simulink library "GenericTarget"  (R2025b)
settings: Solver=VariableStepAuto  StartTime=0.0  StopTime=10.0  RelTol=1e-3
undefined symbols (not defined in the file or in its folder): GT_CheckUniqueParameterValue, strlength
libraries: simulink x4, $bdroot x2, etargetslib x1
(part 2 of 3)

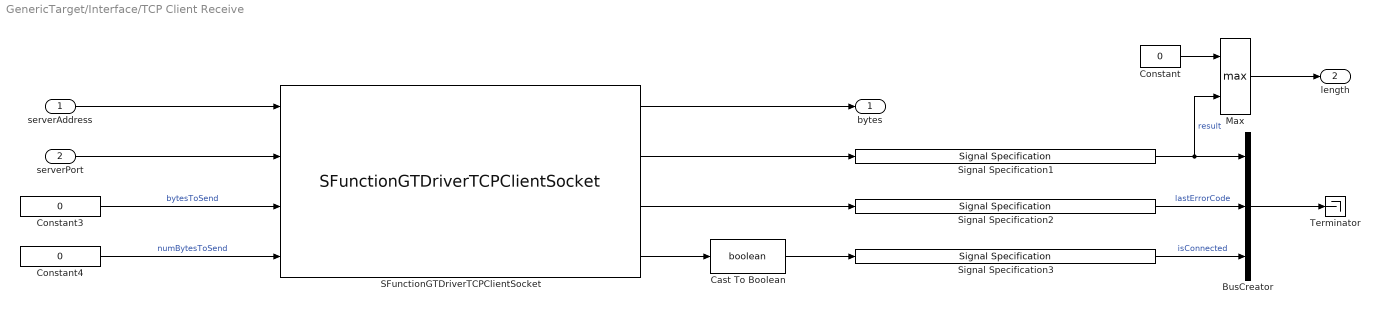
== system GenericTarget/Interface/TCP Client Receive ==
  serverAddress : Inport  OutDataTypeStr=uint8  PortDimensions=4
  serverPort : Inport  Port=2  OutDataTypeStr=uint16  PortDimensions=1
  BusCreator : BusCreator  Inputs=3
  Cast To Boolean : DataTypeConversion  OutDataTypeStr=boolean  SaturateOnIntegerOverflow=off  RndMeth=Floor
  Constant : Constant  Value=0  OutDataTypeStr=int32
  Constant3 : Constant  Value=0  OutDataTypeStr=uint8
  Constant4 : Constant  Value=0  OutDataTypeStr=int32
  Max : MinMax  Function=max  Inputs=2  OutDataTypeStr=int32
  SFunctionGTDriverTCPClientSocket : S-Function  FunctionName=SFunctionGTDriverTCPClientSocket  Parameters=SParameter1, SParameter2, SParameter3, SParameter4, SParameter5, SParameter6, SParameter7, SampleTime  SFunctionDeploymentMode=off  EnableBusSupport=off  mask(Legacy Function){SFunctionSpec=void GT_DriverTCPClientSocketStep(int32 p1, uint8 p5, int32 p6, uint8 y1[p6], int32 y2[1], int32 y3[1], uint8 y4[1], uint8 u1[4], uint16 u2, uint8 p7, uint8 u3[], int32 u4), SParameter1=int32(reshape(localPort, [1 1])), SParameter2=[uint8(deviceName),uint8(0)], SParameter3=uint32(numel(deviceName)), SParameter4=int32(reshape(socketPriority, [1 1])), SParameter5=uint8(0), SParameter6=int32(reshape(rxBufferSize, [1 1])), SParameter7=uint8(reshape(manageConnection, [1 1])), SampleTime=SampleTime, ShowSpec=on}
      mask prompts: SParameter1 "P1:"; SParameter2 "P2:"; SParameter3 "P3:"; SParameter4 "P4:"; SParameter5 "P5:"; SParameter6 "P6:"; SParameter7 "P7:"; SampleTime "Sample time (-1 for inherited):"; ShowSpec "Display function specification"
      mask help:
      | This block allows you to call the legacy functions specified by the following Legacy Code Tool definition:
      | def.SFunctionName = 'SFunctionGTDriverTCPClientSocket';
      | def.OutputFcnSpec = 'void GT_DriverTCPClientSocketStep(int32 p1, uint8 p5, int32 p6, uint8 y1[p6], int32 y2[1], int32 y3[1], uint8 y4[1], uint8 u1[4], uint16 u2, uint8 p7, uint8 u3[], int32 u4)';
      | def.StartFcnSpec = 'void GT_DriverTCPClientSocketInitialize(int32 p1, uint8 p2[], uint32 p3, int32 p4)';
      | def.TerminateFcnSpec = 'void GT_DriverTCPClientSocketTerminate(int32 p1)';
      | def.HeaderFiles = {'GT_DriverTCPClientSocket.hpp'};
      | def.SourceFiles = {'GT_DriverTCPClientSocket.cpp', 'GT_DriverImplementationDetails.cpp'};
      | def.SampleTime = 'parameterized';
      | def.Options.useTlcWithAccel = false;
      | def.Options.language = 'C++';
      mask Help: <p>This block was generated automatically by the Legacy Code Tool. For detailed help on this tool, call<a href="matlab:legacy_code('help')"> legacy_code('help')</a>.</p>
      mask Callback ShowSpec:
      | if strcmp(get_param(gcbh, 'ShowSpec'), 'on')
      |   set_param(gcbh, 'MaskDisplay', sprintf('fprintf(''%s'');', get_param(gcbh, 'SFunctionSpec')));
      | else
      |   set_param(gcbh, 'MaskDisplay', sprintf('fprintf(''%s'');', get_param(gcbh, 'FunctionName')));
      | end
      mask Display: fprintf('void GT_DriverTCPClientSocketStep(int32 p1, uint8 p5, int32 p6, uint8 y1[p6], int32 y2[1], int32 y3[1], uint8 y4[1], uint8 u1[4], uint16 u2, uint8 p7, uint8 u3[], int32 u4)');
  Signal Specification1 : SignalSpecification  OutDataTypeStr=int32  Dimensions=1
  Signal Specification2 : SignalSpecification  OutDataTypeStr=int32  Dimensions=1
  Signal Specification3 : SignalSpecification  OutDataTypeStr=boolean  Dimensions=1
  Terminator : Terminator
  bytes : Outport  OutDataTypeStr=uint8
  length : Outport  Port=2  OutDataTypeStr=int32  PortDimensions=1
  wires:
  Signal Specification2/1 -> BusCreator/2  "lastErrorCode"
  Signal Specification3/1 -> BusCreator/3  "isConnected"
  SFunctionGTDriverTCPClientSocket/1 -> bytes/1
  Constant3/1 -> SFunctionGTDriverTCPClientSocket/3  "bytesToSend"
  Constant4/1 -> SFunctionGTDriverTCPClientSocket/4  "numBytesToSend"
  serverPort/1 -> SFunctionGTDriverTCPClientSocket/2
  serverAddress/1 -> SFunctionGTDriverTCPClientSocket/1
  Cast To Boolean/1 -> Signal Specification3/1
  SFunctionGTDriverTCPClientSocket/2 -> Signal Specification1/1
  SFunctionGTDriverTCPClientSocket/3 -> Signal Specification2/1
  SFunctionGTDriverTCPClientSocket/4 -> Cast To Boolean/1
  Max/1 -> length/1
  Constant/1 -> Max/1
  Signal Specification1/1 -> Max/2, BusCreator/1  "result"
  BusCreator/1 -> Terminator/1

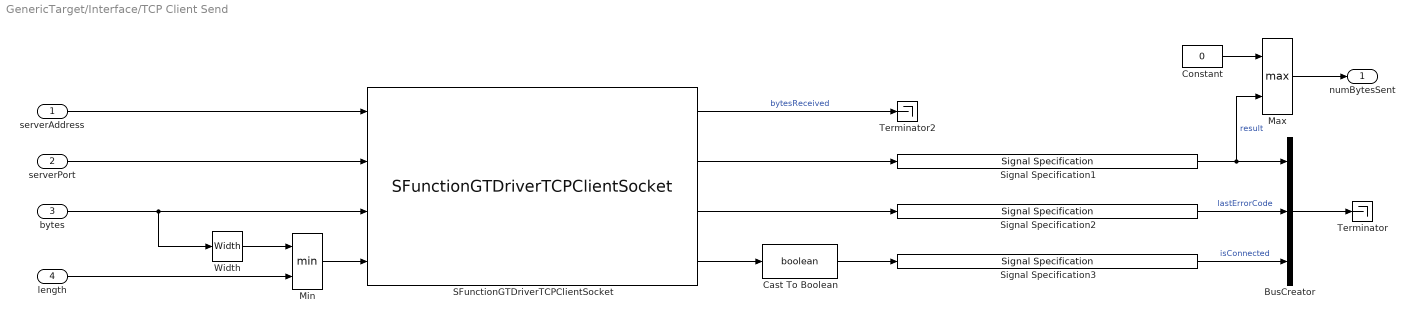
== system GenericTarget/Interface/TCP Client Send ==
  serverAddress : Inport  OutDataTypeStr=uint8  PortDimensions=4
  serverPort : Inport  Port=2  OutDataTypeStr=uint16  PortDimensions=1
  bytes : Inport  Port=3  OutDataTypeStr=uint8
  length : Inport  Port=4  OutDataTypeStr=int32  PortDimensions=1
  BusCreator : BusCreator  Inputs=3
  Cast To Boolean : DataTypeConversion  OutDataTypeStr=boolean  SaturateOnIntegerOverflow=off  RndMeth=Floor
  Constant : Constant  Value=0  OutDataTypeStr=int32
  Max : MinMax  Function=max  Inputs=2  OutDataTypeStr=int32
  Min : MinMax  Inputs=2  OutDataTypeStr=int32
  SFunctionGTDriverTCPClientSocket : S-Function  FunctionName=SFunctionGTDriverTCPClientSocket  Parameters=SParameter1, SParameter2, SParameter3, SParameter4, SParameter5, SParameter6, SParameter7, SampleTime  SFunctionDeploymentMode=off  EnableBusSupport=off  mask(Legacy Function){SFunctionSpec=void GT_DriverTCPClientSocketStep(int32 p1, uint8 p5, int32 p6, uint8 y1[p6], int32 y2[1], int32 y3[1], uint8 y4[1], uint8 u1[4], uint16 u2, uint8 p7, uint8 u3[], int32 u4), SParameter1=int32(reshape(localPort, [1 1])), SParameter2=[uint8(deviceName),uint8(0)], SParameter3=uint32(numel(deviceName)), SParameter4=int32(reshape(socketPriority, [1 1])), SParameter5=uint8(1), SParameter6=int32(1), SParameter7=uint8(reshape(manageConnection, [1 1])), SampleTime=SampleTime, ShowSpec=on}
      mask prompts: SParameter1 "P1:"; SParameter2 "P2:"; SParameter3 "P3:"; SParameter4 "P4:"; SParameter5 "P5:"; SParameter6 "P6:"; SParameter7 "P7:"; SampleTime "Sample time (-1 for inherited):"; ShowSpec "Display function specification"
      mask help:
      | This block allows you to call the legacy functions specified by the following Legacy Code Tool definition:
      | def.SFunctionName = 'SFunctionGTDriverTCPClientSocket';
      | def.OutputFcnSpec = 'void GT_DriverTCPClientSocketStep(int32 p1, uint8 p5, int32 p6, uint8 y1[p6], int32 y2[1], int32 y3[1], uint8 y4[1], uint8 u1[4], uint16 u2, uint8 p7, uint8 u3[], int32 u4)';
      | def.StartFcnSpec = 'void GT_DriverTCPClientSocketInitialize(int32 p1, uint8 p2[], uint32 p3, int32 p4)';
      | def.TerminateFcnSpec = 'void GT_DriverTCPClientSocketTerminate(int32 p1)';
      | def.HeaderFiles = {'GT_DriverTCPClientSocket.hpp'};
      | def.SourceFiles = {'GT_DriverTCPClientSocket.cpp', 'GT_DriverImplementationDetails.cpp'};
      | def.SampleTime = 'parameterized';
      | def.Options.useTlcWithAccel = false;
      | def.Options.language = 'C++';
      mask Help: <p>This block was generated automatically by the Legacy Code Tool. For detailed help on this tool, call<a href="matlab:legacy_code('help')"> legacy_code('help')</a>.</p>
      mask Callback ShowSpec:
      | if strcmp(get_param(gcbh, 'ShowSpec'), 'on')
      |   set_param(gcbh, 'MaskDisplay', sprintf('fprintf(''%s'');', get_param(gcbh, 'SFunctionSpec')));
      | else
      |   set_param(gcbh, 'MaskDisplay', sprintf('fprintf(''%s'');', get_param(gcbh, 'FunctionName')));
      | end
      mask Display: fprintf('void GT_DriverTCPClientSocketStep(int32 p1, uint8 p5, int32 p6, uint8 y1[p6], int32 y2[1], int32 y3[1], uint8 y4[1], uint8 u1[4], uint16 u2, uint8 p7, uint8 u3[], int32 u4)');
  Signal Specification1 : SignalSpecification  OutDataTypeStr=int32  Dimensions=1
  Signal Specification2 : SignalSpecification  OutDataTypeStr=int32  Dimensions=1
  Signal Specification3 : SignalSpecification  OutDataTypeStr=boolean  Dimensions=1
  Terminator : Terminator
  Terminator2 : Terminator
  Width : Width  DataType=int32
  numBytesSent : Outport  OutDataTypeStr=int32  PortDimensions=1
  wires:
  serverAddress/1 -> SFunctionGTDriverTCPClientSocket/1
  serverPort/1 -> SFunctionGTDriverTCPClientSocket/2
  bytes/1 -> SFunctionGTDriverTCPClientSocket/3, Width/1
  Width/1 -> Min/1
  length/1 -> Min/2
  Min/1 -> SFunctionGTDriverTCPClientSocket/4
  SFunctionGTDriverTCPClientSocket/1 -> Terminator2/1  "bytesReceived"
  SFunctionGTDriverTCPClientSocket/2 -> Signal Specification1/1
  SFunctionGTDriverTCPClientSocket/3 -> Signal Specification2/1
  SFunctionGTDriverTCPClientSocket/4 -> Cast To Boolean/1
  Signal Specification1/1 -> Max/2, BusCreator/1  "result"
  Signal Specification2/1 -> BusCreator/2  "lastErrorCode"
  Signal Specification3/1 -> BusCreator/3  "isConnected"
  Cast To Boolean/1 -> Signal Specification3/1
  Constant/1 -> Max/1
  Max/1 -> numBytesSent/1
  BusCreator/1 -> Terminator/1

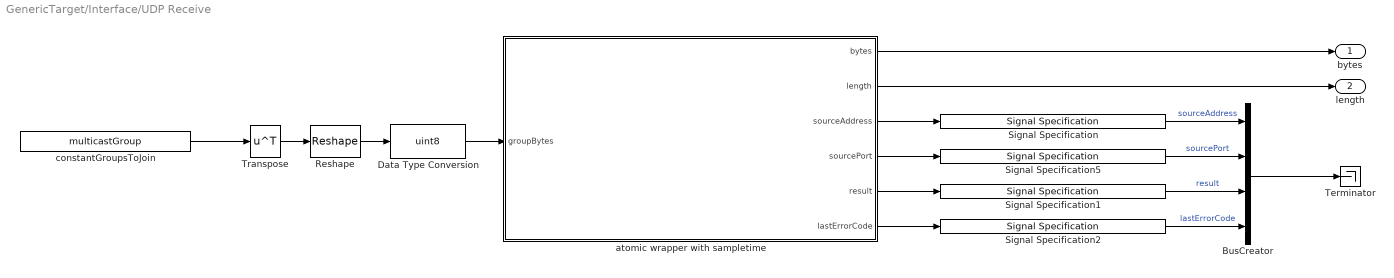
== system GenericTarget/Interface/UDP Receive ==
  BusCreator : BusCreator  Inputs=4
  Data Type Conversion : DataTypeConversion  OutDataTypeStr=uint8  SaturateOnIntegerOverflow=off  RndMeth=Floor
  Reshape : Reshape
  Signal Specification : SignalSpecification  OutDataTypeStr=uint8  Dimensions=4
  Signal Specification1 : SignalSpecification  OutDataTypeStr=int32  Dimensions=1
  Signal Specification2 : SignalSpecification  OutDataTypeStr=int32  Dimensions=1
  Signal Specification5 : SignalSpecification  OutDataTypeStr=uint16  Dimensions=1
  Terminator : Terminator
  Transpose : Math  Operator=transpose
  atomic wrapper with sampletime : Subsystem  TreatAsAtomicUnit=on  SystemSampleTime=SampleTime
  constantGroupsToJoin : Constant  Value=multicastGroup
  bytes : Outport  OutDataTypeStr=uint8  PortDimensions=rxBufferSize
  length : Outport  Port=2  OutDataTypeStr=int32  PortDimensions=1
  wires:
  Signal Specification1/1 -> BusCreator/3  "result"
  Signal Specification2/1 -> BusCreator/4  "lastErrorCode"
  Signal Specification/1 -> BusCreator/1  "sourceAddress"
  Signal Specification5/1 -> BusCreator/2  "sourcePort"
  Transpose/1 -> Reshape/1
  Reshape/1 -> Data Type Conversion/1
  atomic wrapper with sampletime/1(bytes) -> bytes/1
  atomic wrapper with sampletime/2(length) -> length/1
  atomic wrapper with sampletime/3(sourceAddress) -> Signal Specification/1
  atomic wrapper with sampletime/4(sourcePort) -> Signal Specification5/1
  atomic wrapper with sampletime/5(result) -> Signal Specification1/1
  atomic wrapper with sampletime/6(lastErrorCode) -> Signal Specification2/1
  Data Type Conversion/1 -> atomic wrapper with sampletime/1(groupBytes)
  BusCreator/1 -> Terminator/1
  constantGroupsToJoin/1 -> Transpose/1

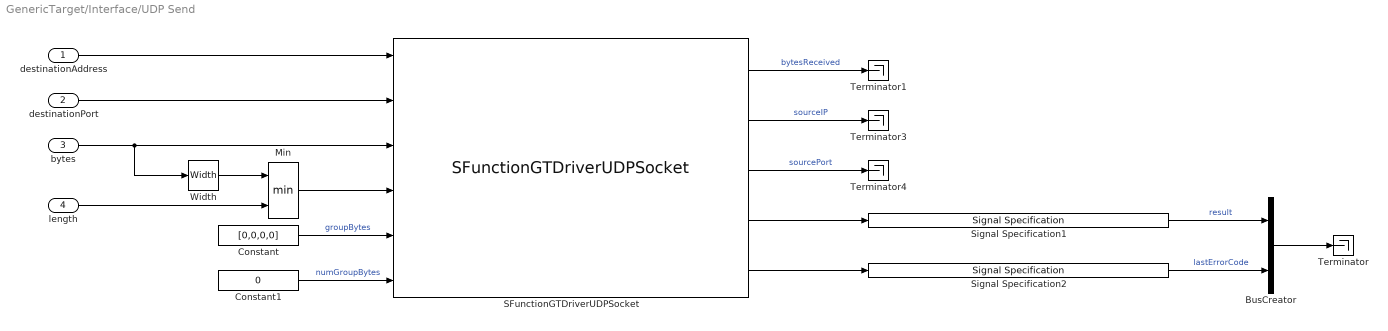
== system GenericTarget/Interface/UDP Send ==
  destinationAddress : Inport  OutDataTypeStr=uint8  PortDimensions=4
  destinationPort : Inport  Port=2  OutDataTypeStr=uint16  PortDimensions=1
  bytes : Inport  Port=3  OutDataTypeStr=uint8
  length : Inport  Port=4  OutDataTypeStr=int32  PortDimensions=1
  BusCreator : BusCreator  Inputs=2
  Constant : Constant  Value=[0,0,0,0]  OutDataTypeStr=uint8
  Constant1 : Constant  Value=0  OutDataTypeStr=uint32
  Min : MinMax  Inputs=2  OutDataTypeStr=int32
  SFunctionGTDriverUDPSocket : S-Function  FunctionName=SFunctionGTDriverUDPSocket  Parameters=SParameter1, SParameter2, SParameter3, SParameter4, SParameter5, SParameter6, SParameter7, SParameter8, SParameter9, SParameter10, SParameter11, SParameter12, SampleTime  SFunctionDeploymentMode=off  EnableBusSupport=off  mask(Legacy Function){SFunctionSpec=void GT_DriverUDPSocketStep(int32 p1, uint8 p11, int32 p12, uint8 y1[p12], uint8 y2[4], uint16 y3[1], int32 y4[1], int32 y5[1], uint8 u1[4], uint16 u2, uint8 u3[], int32 u4, uint8 u5[], uint32 u6), SParameter1=int32(reshape(localPort, [1 1])), SParameter2=[uint8(deviceName),uint8(0)], SParameter3=uint32(numel(deviceName)), SParameter4=int32(reshape(socketPriority, [1 1])), SParameter5=uint8(reshape(allowBroadcast, [1 1])), SParameter6=uint8(reshape(allowZeroLengthMessage, [1 1])), SParameter7=uint8(reshape(multicastAll, [1 1])), SParameter8=uint8(reshape(multicastLoop, [1 1])), SParameter9=uint8(reshape(multicastTTL, [1 1])), SParameter10=uint8(reshape(multicastInterfaceAddress, [1 4])), SParameter11=uint8(1), SParameter12=int32(1), SampleTime=SampleTime, ShowSpec=off}
      mask prompts: SParameter1 "P1:"; SParameter2 "P2:"; SParameter3 "P3:"; SParameter4 "P4:"; SParameter5 "P5:"; SParameter6 "P6:"; SParameter7 "P7:"; SParameter8 "P8:"; SParameter9 "P9:"; SParameter10 "P10:"; SParameter11 "P11:"; SParameter12 "P12:"; SampleTime "Sample time (-1 for inherited):"; ShowSpec "Display function specification"
      mask help:
      | This block allows you to call the legacy functions specified by the following Legacy Code Tool definition:
      | def.SFunctionName = 'SFunctionGTDriverUDPSocket';
      | def.OutputFcnSpec = 'void GT_DriverUDPSocketStep(int32 p1, uint8 p11, int32 p12, uint8 y1[p12], uint8 y2[4], uint16 y3[1], int32 y4[1], int32 y5[1], uint8 u1[4], uint16 u2, uint8 u3[], int32 u4, uint8 u5[], uint32 u6)';
      | def.StartFcnSpec = 'void GT_DriverUDPSocketInitialize(int32 p1, uint8 p2[], uint32 p3, int32 p4, uint8 p5, uint8 p6, uint8 p7, uint8 p8, uint8 p9, uint8 p10[4])';
      | def.TerminateFcnSpec = 'void GT_DriverUDPSocketTerminate(int32 p1)';
      | def.HeaderFiles = {'GT_DriverUDPSocket.hpp'};
      | def.SourceFiles = {'GT_DriverUDPSocket.cpp', 'GT_DriverImplementationDetails.cpp'};
      | def.SampleTime = 'parameterized';
      | def.Options.useTlcWithAccel = false;
      | def.Options.language = 'C++';
      mask Help: <p>This block was generated automatically by the Legacy Code Tool. For detailed help on this tool, call<a href="matlab:legacy_code('help')"> legacy_code('help')</a>.</p>
      mask Callback ShowSpec:
      | if strcmp(get_param(gcbh, 'ShowSpec'), 'on')
      |   set_param(gcbh, 'MaskDisplay', sprintf('fprintf(''%s'');', get_param(gcbh, 'SFunctionSpec')));
      | else
      |   set_param(gcbh, 'MaskDisplay', sprintf('fprintf(''%s'');', get_param(gcbh, 'FunctionName')));
      | end
      mask Display: fprintf('SFunctionGTDriverUDPSocket');
  Signal Specification1 : SignalSpecification  OutDataTypeStr=int32  Dimensions=1
  Signal Specification2 : SignalSpecification  OutDataTypeStr=int32  Dimensions=1
  Terminator{,1,3..4} (4 alike) : Terminator
  Width : Width  DataType=int32
  wires:
  destinationAddress/1 -> SFunctionGTDriverUDPSocket/1
  bytes/1 -> SFunctionGTDriverUDPSocket/3, Width/1
  destinationPort/1 -> SFunctionGTDriverUDPSocket/2
  Min/1 -> SFunctionGTDriverUDPSocket/4
  Width/1 -> Min/1
  length/1 -> Min/2
  Signal Specification1/1 -> BusCreator/1  "result"
  Signal Specification2/1 -> BusCreator/2  "lastErrorCode"
  Constant/1 -> SFunctionGTDriverUDPSocket/5  "groupBytes"
  Constant1/1 -> SFunctionGTDriverUDPSocket/6  "numGroupBytes"
  SFunctionGTDriverUDPSocket/1 -> Terminator1/1  "bytesReceived"
  SFunctionGTDriverUDPSocket/2 -> Terminator3/1  "sourceIP"
  SFunctionGTDriverUDPSocket/3 -> Terminator4/1  "sourcePort"
  SFunctionGTDriverUDPSocket/4 -> Signal Specification1/1
  SFunctionGTDriverUDPSocket/5 -> Signal Specification2/1
  BusCreator/1 -> Terminator/1

== system GenericTarget/Interface/Write Bus To File ==
  bus : Inport
  BusSelector : BusSelector  OutputSignals=a
  BytePack : etargetslib/Byte Pack  datatypes={'double'}  byteAlign=1
  Constant : Constant  Value=0.0  OutDataTypeStr=double
  Digital Clock : DigitalClock  SampleTime=SampleTime
  SFunctionGTDriverDataRecorder : S-Function  FunctionName=SFunctionGTDriverDataRecorder  Parameters=SParameter1, SParameter2, SParameter3, SParameter4, SParameter5, SParameter6, SParameter7, SParameter8, SParameter9, SParameter10, SParameter11, SParameter12, SParameter13, SParameter14, SampleTime  SFunctionDeploymentMode=off  EnableBusSupport=off  mask(Legacy Function){SFunctionSpec=void GT_DriverDataRecorderStep(uint8 p1, uint8 p2[], uint32 p3, double u1, double u2[p6], uint32 p6, uint8 u3[p5], uint32 p5, uint8 p14), SParameter1=uint8(1), SParameter2=uint8(strID), SParameter3=uint32(strlength(strID)), SParameter4=uint32(reshape(numSamplesPerFile, [1 1])), SParameter5=uint32(reshape(numBytesPerSample, [1 1])), SParameter6=uint32(1), SParameter7=uint8(strSignalNames), SParameter8=uint32(reshape(strlenSignalNames, [1 1])), SParameter9=uint8(strDimensions), SParameter10=uint32(reshape(strlenDimensions, [1 1])), SParameter11=uint8(strDataTypes), SParameter12=uint32(reshape(strlenDataTypes, [1 1])), SParameter13=int32(reshape(threadPriority, [1 1])), SParameter14=uint8(reshape(writeFilesDuringSimulation, [1 1])), SampleTime=SampleTime, ShowSpec=on}
      mask prompts: SParameter1 "P1:"; SParameter2 "P2:"; SParameter3 "P3:"; SParameter4 "P4:"; SParameter5 "P5:"; SParameter6 "P6:"; SParameter7 "P7:"; SParameter8 "P8:"; SParameter9 "P9:"; SParameter10 "P10:"; SParameter11 "P11:"; SParameter12 "P12:"; SParameter13 "P13:"; SParameter14 "P14:"; SampleTime "Sample time (-1 for inherited):"; ShowSpec "Display function specification"
      mask help:
      | This block allows you to call the legacy functions specified by the following Legacy Code Tool definition:
      | def.SFunctionName = 'SFunctionGTDriverDataRecorder';
      | def.OutputFcnSpec = 'void GT_DriverDataRecorderStep(uint8 p1, uint8 p2[], uint32 p3, double u1, double u2[p6], uint32 p6, uint8 u3[p5], uint32 p5, uint8 p14)';
      | def.StartFcnSpec = 'void GT_DriverDataRecorderInitialize(uint8 p1, uint8 p2[], uint32 p3, uint32 p4, uint32 p5, uint32 p6, uint8 p7[], uint32 p8, uint8 p9[], uint32 p10, uint8 p11[], uint32 p12, int32 p13, uint8 p14)';
      | def.TerminateFcnSpec = 'void GT_DriverDataRecorderTerminate(uint8 p14)';
      | def.HeaderFiles = {'GT_DriverDataRecorder.hpp'};
      | def.SourceFiles = {'GT_DriverDataRecorder.cpp', 'GT_DriverImplementationDetails.cpp'};
      | def.SampleTime = 'parameterized';
      | def.Options.useTlcWithAccel = false;
      | def.Options.language = 'C++';
      mask Help: <p>This block was generated automatically by the Legacy Code Tool. For detailed help on this tool, call<a href="matlab:legacy_code('help')"> legacy_code('help')</a>.</p>
      mask Callback ShowSpec:
      | if strcmp(get_param(gcbh, 'ShowSpec'), 'on')
      |   set_param(gcbh, 'MaskDisplay', sprintf('fprintf(''%s'');', get_param(gcbh, 'SFunctionSpec')));
      | else
      |   set_param(gcbh, 'MaskDisplay', sprintf('fprintf(''%s'');', get_param(gcbh, 'FunctionName')));
      | end
      mask Display: fprintf('void GT_DriverDataRecorderStep(uint8 p1, uint8 p2[], uint32 p3, double u1, double u2[p6], uint32 p6, uint8 u3[p5], uint32 p5, uint8 p14)');
  wires:
  BytePack/1 -> SFunctionGTDriverDataRecorder/3
  bus/1 -> BusSelector/1
  Digital Clock/1 -> SFunctionGTDriverDataRecorder/1
  Constant/1 -> SFunctionGTDriverDataRecorder/2
  BusSelector/1 -> BytePack/1  "<a>"

== system GenericTarget/Interface/Write Scalar Doubles To File ==
  bus : Inport
  Bus to Vector : BusToVector
  BusSelector : BusSelector  OutputSignals=signal1,signal2  OutputAsBus=on
  Constant : Constant  Value=0  OutDataTypeStr=uint8
  Digital Clock : DigitalClock  SampleTime=SampleTime
  SFunctionGTDriverDataRecorder : S-Function  FunctionName=SFunctionGTDriverDataRecorder  Parameters=SParameter1, SParameter2, SParameter3, SParameter4, SParameter5, SParameter6, SParameter7, SParameter8, SParameter9, SParameter10, SParameter11, SParameter12, SParameter13, SParameter14, SampleTime  SFunctionDeploymentMode=off  EnableBusSupport=off  mask(Legacy Function){SFunctionSpec=void GT_DriverDataRecorderStep(uint8 p1, uint8 p2[], uint32 p3, double u1, double u2[p6], uint32 p6, uint8 u3[p5], uint32 p5, uint8 p14), SParameter1=uint8(0), SParameter2=uint8(strID), SParameter3=uint32(strlength(strID)), SParameter4=uint32(reshape(numSamplesPerFile, [1 1])), SParameter5=uint32(1), SParameter6=uint32(reshape(numSignals, [1 1])), SParameter7=uint8(signalNames), SParameter8=uint32(reshape(numCharacters, [1 1])), SParameter9=uint8(ones([1 1 ])), SParameter10=uint32(0), SParameter11=uint8(ones([1 1 ])), SParameter12=uint32(0), SParameter13=int32(reshape(threadPriority, [1 1])), SParameter14=uint8(reshape(writeFilesDuringSimulation, [1 1])), SampleTime=SampleTime, ShowSpec=on}
      mask prompts: SParameter1 "P1:"; SParameter2 "P2:"; SParameter3 "P3:"; SParameter4 "P4:"; SParameter5 "P5:"; SParameter6 "P6:"; SParameter7 "P7:"; SParameter8 "P8:"; SParameter9 "P9:"; SParameter10 "P10:"; SParameter11 "P11:"; SParameter12 "P12:"; SParameter13 "P13:"; SParameter14 "P14:"; SampleTime "Sample time (-1 for inherited):"; ShowSpec "Display function specification"
      mask help:
      | This block allows you to call the legacy functions specified by the following Legacy Code Tool definition:
      | def.SFunctionName = 'SFunctionGTDriverDataRecorder';
      | def.OutputFcnSpec = 'void GT_DriverDataRecorderStep(uint8 p1, uint8 p2[], uint32 p3, double u1, double u2[p6], uint32 p6, uint8 u3[p5], uint32 p5, uint8 p14)';
      | def.StartFcnSpec = 'void GT_DriverDataRecorderInitialize(uint8 p1, uint8 p2[], uint32 p3, uint32 p4, uint32 p5, uint32 p6, uint8 p7[], uint32 p8, uint8 p9[], uint32 p10, uint8 p11[], uint32 p12, int32 p13, uint8 p14)';
      | def.TerminateFcnSpec = 'void GT_DriverDataRecorderTerminate(uint8 p14)';
      | def.HeaderFiles = {'GT_DriverDataRecorder.hpp'};
      | def.SourceFiles = {'GT_DriverDataRecorder.cpp', 'GT_DriverImplementationDetails.cpp'};
      | def.SampleTime = 'parameterized';
      | def.Options.useTlcWithAccel = false;
      | def.Options.language = 'C++';
      mask Help: <p>This block was generated automatically by the Legacy Code Tool. For detailed help on this tool, call<a href="matlab:legacy_code('help')"> legacy_code('help')</a>.</p>
      mask Callback ShowSpec:
      | if strcmp(get_param(gcbh, 'ShowSpec'), 'on')
      |   set_param(gcbh, 'MaskDisplay', sprintf('fprintf(''%s'');', get_param(gcbh, 'SFunctionSpec')));
      | else
      |   set_param(gcbh, 'MaskDisplay', sprintf('fprintf(''%s'');', get_param(gcbh, 'FunctionName')));
      | end
      mask Display: fprintf('void GT_DriverDataRecorderStep(uint8 p1, uint8 p2[], uint32 p3, double u1, double u2[p6], uint32 p6, uint8 u3[p5], uint32 p5, uint8 p14)');
  wires:
  bus/1 -> BusSelector/1
  BusSelector/1 -> Bus to Vector/1
  Digital Clock/1 -> SFunctionGTDriverDataRecorder/1
  Bus to Vector/1 -> SFunctionGTDriverDataRecorder/2
  Constant/1 -> SFunctionGTDriverDataRecorder/3

== system GenericTarget/Target Stats/Application Arguments ==
  Reshape : Reshape  OutputDimensionality=Customize  OutputDimensions=[maxNumCharsPerArgument,maxNumArguments]
  SFunctionGTDriverApplicationArguments : S-Function  FunctionName=SFunctionGTDriverApplicationArguments  Parameters=SParameter1, SParameter2, SampleTime  SFunctionDeploymentMode=off  EnableBusSupport=off  mask(Legacy Function){SFunctionSpec=void GT_DriverApplicationArgumentsStep(uint8 y1[p1*p2], uint32 y2[p2], uint32 y3[1], uint32 p1, uint32 p2), SParameter1=uint32(maxNumCharsPerArgument), SParameter2=uint32(maxNumArguments), SampleTime=SampleTime, ShowSpec=on}
      mask prompts: SParameter1 "P1:"; SParameter2 "P2:"; SampleTime "Sample time (-1 for inherited):"; ShowSpec "Display function specification"
      mask help:
      | This block allows you to call the legacy functions specified by the following Legacy Code Tool definition:
      | def.SFunctionName = 'SFunctionGTDriverApplicationArguments';
      | def.OutputFcnSpec = 'void GT_DriverApplicationArgumentsStep(uint8 y1[p1*p2], uint32 y2[p2], uint32 y3[1], uint32 p1, uint32 p2)';
      | def.StartFcnSpec = 'void GT_DriverApplicationArgumentsInitialize()';
      | def.TerminateFcnSpec = 'void GT_DriverApplicationArgumentsTerminate()';
      | def.HeaderFiles = {'GT_DriverApplicationArguments.hpp'};
      | def.SourceFiles = {'GT_DriverApplicationArguments.cpp'};
      | def.SampleTime = 'parameterized';
      | def.Options.useTlcWithAccel = false;
      | def.Options.language = 'C++';
      mask Help: <p>This block was generated automatically by the Legacy Code Tool. For detailed help on this tool, call<a href="matlab:legacy_code('help')"> legacy_code('help')</a>.</p>
      mask Callback ShowSpec:
      | if strcmp(get_param(gcbh, 'ShowSpec'), 'on')
      |   set_param(gcbh, 'MaskDisplay', sprintf('fprintf(''%s'');', get_param(gcbh, 'SFunctionSpec')));
      | else
      |   set_param(gcbh, 'MaskDisplay', sprintf('fprintf(''%s'');', get_param(gcbh, 'FunctionName')));
      | end
      mask Display: fprintf('void GT_DriverApplicationArgumentsStep(uint8 y1[p1*p2], uint32 y2[p2], uint32 y3[1], uint32 p1, uint32 p2)');
  args : Outport  OutDataTypeStr=uint8  PortDimensions=[maxNumCharsPerArgument,maxNumArguments]
  numCharacters : Outport  Port=2  OutDataTypeStr=uint32  PortDimensions=maxNumArguments
  numArguments : Outport  Port=3  OutDataTypeStr=uint32  PortDimensions=1
  wires:
  SFunctionGTDriverApplicationArguments/1 -> Reshape/1
  SFunctionGTDriverApplicationArguments/2 -> numCharacters/1
  SFunctionGTDriverApplicationArguments/3 -> numArguments/1
  Reshape/1 -> args/1

== system GenericTarget/Target Stats/Read Thermal Zones ==
  SFunctionGTDriverReadThermalZones : S-Function  FunctionName=SFunctionGTDriverReadThermalZones  Parameters=SParameter1, SampleTime  SFunctionDeploymentMode=off  EnableBusSupport=off  mask(Legacy Function){SFunctionSpec=void GT_DriverReadThermalZonesStep(uint32 p1, double y1[p1]), SParameter1=uint32(reshape(maxNumThermalZones, [1,1])), SampleTime=SampleTime, ShowSpec=on}
      mask prompts: SParameter1 "P1:"; SampleTime "Sample time (-1 for inherited):"; ShowSpec "Display function specification"
      mask help:
      | This block allows you to call the legacy functions specified by the following Legacy Code Tool definition:
      | def.SFunctionName = 'SFunctionGTDriverReadThermalZones';
      | def.OutputFcnSpec = 'void GT_DriverReadThermalZonesStep(uint32 p1, double y1[p1])';
      | def.StartFcnSpec = 'void GT_DriverReadThermalZonesInitialize()';
      | def.TerminateFcnSpec = 'void GT_DriverReadThermalZonesTerminate()';
      | def.HeaderFiles = {'GT_DriverReadThermalZones.hpp'};
      | def.SourceFiles = {'GT_DriverReadThermalZones.cpp'};
      | def.SampleTime = 'parameterized';
      | def.Options.useTlcWithAccel = false;
      | def.Options.language = 'C++';
      mask Help: <p>This block was generated automatically by the Legacy Code Tool. For detailed help on this tool, call<a href="matlab:legacy_code('help')"> legacy_code('help')</a>.</p>
      mask Callback ShowSpec:
      | if strcmp(get_param(gcbh, 'ShowSpec'), 'on')
      |   set_param(gcbh, 'MaskDisplay', sprintf('fprintf(''%s'');', get_param(gcbh, 'SFunctionSpec')));
      | else
      |   set_param(gcbh, 'MaskDisplay', sprintf('fprintf(''%s'');', get_param(gcbh, 'FunctionName')));
      | end
      mask Display: fprintf('void GT_DriverReadThermalZonesStep(uint32 p1, double y1[p1])');
  Signal Specification : SignalSpecification  OutDataTypeStr=double  Unit=°C  Dimensions=maxNumThermalZones
  temperatures : Outport
  wires:
  SFunctionGTDriverReadThermalZones/1 -> Signal Specification/1
  Signal Specification/1 -> temperatures/1

== system GenericTarget/Time/CPU Overloads ==
  SFunctionGTDriverNumCPUOverloads : S-Function  FunctionName=SFunctionGTDriverNumCPUOverloads  Parameters=SampleTime  SFunctionDeploymentMode=off  EnableBusSupport=off  mask(Legacy Function){SFunctionSpec=void GT_DriverNumCPUOverloadsStep(uint64 y1[1], uint64 y2[1]), SampleTime=SampleTime, ShowSpec=on}
      mask prompts: SampleTime "Sample time (-1 for inherited):"; ShowSpec "Display function specification"
      mask help:
      | This block allows you to call the legacy functions specified by the following Legacy Code Tool definition:
      | def.SFunctionName = 'SFunctionGTDriverNumCPUOverloads';
      | def.OutputFcnSpec = 'void GT_DriverNumCPUOverloadsStep(uint64 y1[1], uint64 y2[1])';
      | def.StartFcnSpec = 'void GT_DriverNumCPUOverloadsInitialize()';
      | def.TerminateFcnSpec = 'void GT_DriverNumCPUOverloadsTerminate()';
      | def.HeaderFiles = {'GT_DriverNumCPUOverloads.hpp'};
      | def.SourceFiles = {'GT_DriverNumCPUOverloads.cpp'};
      | def.SampleTime = 'parameterized';
      | def.Options.useTlcWithAccel = false;
      | def.Options.language = 'C++';
      mask Help: <p>This block was generated automatically by the Legacy Code Tool. For detailed help on this tool, call<a href="matlab:legacy_code('help')"> legacy_code('help')</a>.</p>
      mask Callback ShowSpec:
      | if strcmp(get_param(gcbh, 'ShowSpec'), 'on')
      |   set_param(gcbh, 'MaskDisplay', sprintf('fprintf(''%s'');', get_param(gcbh, 'SFunctionSpec')));
      | else
      |   set_param(gcbh, 'MaskDisplay', sprintf('fprintf(''%s'');', get_param(gcbh, 'FunctionName')));
      | end
      mask Display: fprintf('void GT_DriverNumCPUOverloadsStep(uint64 y1[1], uint64 y2[1])');
  numCPUOverloads : Outport  OutDataTypeStr=uint64  PortDimensions=1
  numLostTicks : Outport  Port=2  OutDataTypeStr=uint64  PortDimensions=1
  wires:
  SFunctionGTDriverNumCPUOverloads/1 -> numCPUOverloads/1
  SFunctionGTDriverNumCPUOverloads/2 -> numLostTicks/1

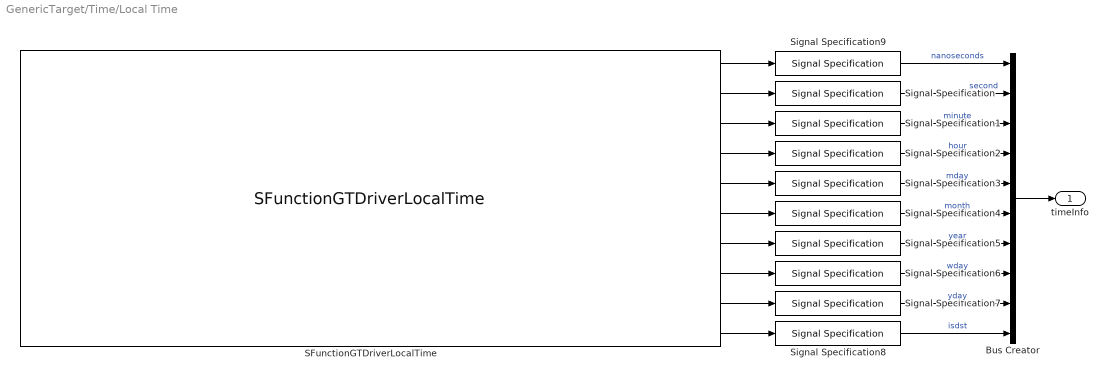
== system GenericTarget/Time/Local Time ==
  Bus Creator : BusCreator  Inputs=10
  SFunctionGTDriverLocalTime : S-Function  FunctionName=SFunctionGTDriverLocalTime  Parameters=SampleTime  SFunctionDeploymentMode=off  EnableBusSupport=off  mask(Legacy Function){SFunctionSpec=void GT_DriverLocalTimeStep(int32 y1[1], int32 y2[1], int32 y3[1], int32 y4[1], int32 y5[1], int32 y6[1], int32 y7[1], int32 y8[1], int32 y9[1], int32 y10[1]), SampleTime=SampleTime, ShowSpec=on}
      mask prompts: SampleTime "Sample time (-1 for inherited):"; ShowSpec "Display function specification"
      mask help:
      | This block allows you to call the legacy functions specified by the following Legacy Code Tool definition:
      | def.SFunctionName = 'SFunctionGTDriverLocalTime';
      | def.OutputFcnSpec = 'void GT_DriverLocalTimeStep(int32 y1[1], int32 y2[1], int32 y3[1], int32 y4[1], int32 y5[1], int32 y6[1], int32 y7[1], int32 y8[1], int32 y9[1], int32 y10[1])';
      | def.StartFcnSpec = 'void GT_DriverLocalTimeInitialize()';
      | def.TerminateFcnSpec = 'void GT_DriverLocalTimeTerminate()';
      | def.HeaderFiles = {'GT_DriverLocalTime.hpp'};
      | def.SourceFiles = {'GT_DriverLocalTime.cpp'};
      | def.SampleTime = 'parameterized';
      | def.Options.useTlcWithAccel = false;
      | def.Options.language = 'C++';
      mask Help: <p>This block was generated automatically by the Legacy Code Tool. For detailed help on this tool, call<a href="matlab:legacy_code('help')"> legacy_code('help')</a>.</p>
      mask Callback ShowSpec:
      | if strcmp(get_param(gcbh, 'ShowSpec'), 'on')
      |   set_param(gcbh, 'MaskDisplay', sprintf('fprintf(''%s'');', get_param(gcbh, 'SFunctionSpec')));
      | else
      |   set_param(gcbh, 'MaskDisplay', sprintf('fprintf(''%s'');', get_param(gcbh, 'FunctionName')));
      | end
      mask Display: fprintf('void GT_DriverLocalTimeStep(int32 y1[1], int32 y2[1], int32 y3[1], int32 y4[1], int32 y5[1], int32 y6[1], int32 y7[1], int32 y8[1], int32 y9[1], int32 y10[1])');
  Signal Specification : SignalSpecification  OutDataTypeStr=int32  Unit=s  Dimensions=1
  Signal Specification1 : SignalSpecification  OutDataTypeStr=int32  Unit=min  Dimensions=1
  Signal Specification2 : SignalSpecification  OutDataTypeStr=int32  Unit=h  Dimensions=1
  Signal Specification3 : SignalSpecification  OutDataTypeStr=int32  Unit=d  Dimensions=1
  Signal Specification4 : SignalSpecification  OutDataTypeStr=int32  Dimensions=1
  Signal Specification5 : SignalSpecification  OutDataTypeStr=int32  Dimensions=1
  Signal Specification6 : SignalSpecification  OutDataTypeStr=int32  Unit=d  Dimensions=1
  Signal Specification7 : SignalSpecification  OutDataTypeStr=int32  Unit=d  Dimensions=1
  Signal Specification8 : SignalSpecification  OutDataTypeStr=int32  Dimensions=1
  Signal Specification9 : SignalSpecification  OutDataTypeStr=int32  Unit=ns  Dimensions=1
  timeInfo : Outport  VectorParamsAs1DForOutWhenUnconnected=off
  wires:
  Signal Specification/1 -> Bus Creator/2  "second"
  Signal Specification3/1 -> Bus Creator/5  "mday"
  Signal Specification4/1 -> Bus Creator/6  "month"
  Signal Specification1/1 -> Bus Creator/3  "minute"
  Signal Specification2/1 -> Bus Creator/4  "hour"
  Bus Creator/1 -> timeInfo/1
  Signal Specification5/1 -> Bus Creator/7  "year"
  Signal Specification6/1 -> Bus Creator/8  "wday"
  Signal Specification7/1 -> Bus Creator/9  "yday"
  Signal Specification8/1 -> Bus Creator/10  "isdst"
  Signal Specification9/1 -> Bus Creator/1  "nanoseconds"
  SFunctionGTDriverLocalTime/1 -> Signal Specification9/1
  SFunctionGTDriverLocalTime/2 -> Signal Specification/1
  SFunctionGTDriverLocalTime/3 -> Signal Specification1/1
  SFunctionGTDriverLocalTime/4 -> Signal Specification2/1
  SFunctionGTDriverLocalTime/5 -> Signal Specification3/1
  SFunctionGTDriverLocalTime/6 -> Signal Specification4/1
  SFunctionGTDriverLocalTime/7 -> Signal Specification5/1
  SFunctionGTDriverLocalTime/8 -> Signal Specification6/1
  SFunctionGTDriverLocalTime/9 -> Signal Specification7/1
  SFunctionGTDriverLocalTime/10 -> Signal Specification8/1

== system GenericTarget/Time/Model Execution Time ==
  SFunctionGTDriverModelExecutionTime : S-Function  FunctionName=SFunctionGTDriverModelExecutionTime  Parameters=SampleTime  SFunctionDeploymentMode=off  EnableBusSupport=off  mask(Legacy Function){SFunctionSpec=void GT_DriverModelExecutionTimeStep(double y1[1]), SampleTime=SampleTime, ShowSpec=on}
      mask prompts: SampleTime "Sample time (-1 for inherited):"; ShowSpec "Display function specification"
      mask help:
      | This block allows you to call the legacy functions specified by the following Legacy Code Tool definition:
      | def.SFunctionName = 'SFunctionGTDriverModelExecutionTime';
      | def.OutputFcnSpec = 'void GT_DriverModelExecutionTimeStep(double y1[1])';
      | def.StartFcnSpec = 'void GT_DriverModelExecutionTimeInitialize()';
      | def.TerminateFcnSpec = 'void GT_DriverModelExecutionTimeTerminate()';
      | def.HeaderFiles = {'GT_DriverModelExecutionTime.hpp'};
      | def.SourceFiles = {'GT_DriverModelExecutionTime.cpp'};
      | def.SampleTime = 'parameterized';
      | def.Options.useTlcWithAccel = false;
      | def.Options.language = 'C++';
      mask Help: <p>This block was generated automatically by the Legacy Code Tool. For detailed help on this tool, call<a href="matlab:legacy_code('help')"> legacy_code('help')</a>.</p>
      mask Callback ShowSpec:
      | if strcmp(get_param(gcbh, 'ShowSpec'), 'on')
      |   set_param(gcbh, 'MaskDisplay', sprintf('fprintf(''%s'');', get_param(gcbh, 'SFunctionSpec')));
      | else
      |   set_param(gcbh, 'MaskDisplay', sprintf('fprintf(''%s'');', get_param(gcbh, 'FunctionName')));
      | end
      mask Display: fprintf('void GT_DriverModelExecutionTimeStep(double y1[1])');
  time : Outport  OutDataTypeStr=double  Unit=s  PortDimensions=1  VectorParamsAs1DForOutWhenUnconnected=off
  wires:
  SFunctionGTDriverModelExecutionTime/1 -> time/1

== system GenericTarget/Time/Task Execution Time ==
  SFunctionGTDriverTaskExecutionTime : S-Function  FunctionName=SFunctionGTDriverTaskExecutionTime  Parameters=SParameter1, SParameter2, SampleTime  SFunctionDeploymentMode=off  EnableBusSupport=off  mask(Legacy Function){SFunctionSpec=void GT_DriverTaskExecutionTimeStep(double y1[1], uint8 p1[], uint32 p2), SParameter1=uint8(strTaskName), SParameter2=uint32(strlength(strTaskName)), SampleTime=SampleTime, ShowSpec=on}
      mask prompts: SParameter1 "P1:"; SParameter2 "P2:"; SampleTime "Sample time (-1 for inherited):"; ShowSpec "Display function specification"
      mask help:
      | This block allows you to call the legacy functions specified by the following Legacy Code Tool definition:
      | def.SFunctionName = 'SFunctionGTDriverTaskExecutionTime';
      | def.OutputFcnSpec = 'void GT_DriverTaskExecutionTimeStep(double y1[1], uint8 p1[], uint32 p2)';
      | def.StartFcnSpec = 'void GT_DriverTaskExecutionTimeInitialize()';
      | def.TerminateFcnSpec = 'void GT_DriverTaskExecutionTimeTerminate()';
      | def.HeaderFiles = {'GT_DriverTaskExecutionTime.hpp'};
      | def.SourceFiles = {'GT_DriverTaskExecutionTime.cpp'};
      | def.SampleTime = 'parameterized';
      | def.Options.useTlcWithAccel = false;
      | def.Options.language = 'C++';
      mask Help: <p>This block was generated automatically by the Legacy Code Tool. For detailed help on this tool, call<a href="matlab:legacy_code('help')"> legacy_code('help')</a>.</p>
      mask Callback ShowSpec:
      | if strcmp(get_param(gcbh, 'ShowSpec'), 'on')
      |   set_param(gcbh, 'MaskDisplay', sprintf('fprintf(''%s'');', get_param(gcbh, 'SFunctionSpec')));
      | else
      |   set_param(gcbh, 'MaskDisplay', sprintf('fprintf(''%s'');', get_param(gcbh, 'FunctionName')));
      | end
      mask Display: fprintf('void GT_DriverTaskExecutionTimeStep(double y1[1], uint8 p1[], uint32 p2)');
  taskExecutionTime : Outport  OutDataTypeStr=double  Unit=s  PortDimensions=1  VectorParamsAs1DForOutWhenUnconnected=off
  wires:
  SFunctionGTDriverTaskExecutionTime/1 -> taskExecutionTime/1

== system GenericTarget/Time/Task Overloads ==
  SFunctionGTDriverNumTaskOverloads : S-Function  FunctionName=SFunctionGTDriverNumTaskOverloads  Parameters=SParameter1, SParameter2, SampleTime  SFunctionDeploymentMode=off  EnableBusSupport=off  mask(Legacy Function){SFunctionSpec=void GT_DriverNumTaskOverloadsStep(uint64 y1[1], uint8 p1[], uint32 p2), SParameter1=uint8(strTaskName), SParameter2=uint32(strlength(strTaskName)), SampleTime=SampleTime, ShowSpec=on}
      mask prompts: SParameter1 "P1:"; SParameter2 "P2:"; SampleTime "Sample time (-1 for inherited):"; ShowSpec "Display function specification"
      mask help:
      | This block allows you to call the legacy functions specified by the following Legacy Code Tool definition:
      | def.SFunctionName = 'SFunctionGTDriverNumTaskOverloads';
      | def.OutputFcnSpec = 'void GT_DriverNumTaskOverloadsStep(uint64 y1[1], uint8 p1[], uint32 p2)';
      | def.StartFcnSpec = 'void GT_DriverNumTaskOverloadsInitialize()';
      | def.TerminateFcnSpec = 'void GT_DriverNumTaskOverloadsTerminate()';
      | def.HeaderFiles = {'GT_DriverNumTaskOverloads.hpp'};
      | def.SourceFiles = {'GT_DriverNumTaskOverloads.cpp'};
      | def.SampleTime = 'parameterized';
      | def.Options.useTlcWithAccel = false;
      | def.Options.language = 'C++';
      mask Help: <p>This block was generated automatically by the Legacy Code Tool. For detailed help on this tool, call<a href="matlab:legacy_code('help')"> legacy_code('help')</a>.</p>
      mask Callback ShowSpec:
      | if strcmp(get_param(gcbh, 'ShowSpec'), 'on')
      |   set_param(gcbh, 'MaskDisplay', sprintf('fprintf(''%s'');', get_param(gcbh, 'SFunctionSpec')));
      | else
      |   set_param(gcbh, 'MaskDisplay', sprintf('fprintf(''%s'');', get_param(gcbh, 'FunctionName')));
      | end
      mask Display: fprintf('void GT_DriverNumTaskOverloadsStep(uint64 y1[1], uint8 p1[], uint32 p2)');
  numTaskOverloads : Outport  OutDataTypeStr=uint64  PortDimensions=1
  wires:
  SFunctionGTDriverNumTaskOverloads/1 -> numTaskOverloads/1

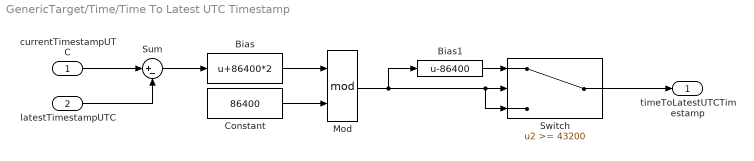
== system GenericTarget/Time/Time To Latest UTC Timestamp ==
  currentTimestampUTC : Inport  Unit=s
  latestTimestampUTC : Inport  Port=2  Unit=s
  Bias : Bias  Bias=86400*2  SaturateOnIntegerOverflow=off
  Bias1 : Bias  Bias=-86400  SaturateOnIntegerOverflow=off
  Constant : Constant  Value=86400
  Mod : Math  Operator=mod  SignedPower=on
  Sum : Sum  Inputs=|+-
  Switch : Switch  Threshold=43200  SaturateOnIntegerOverflow=off  InputSameDT=off
  timeToLatestUTCTimestamp : Outport  Unit=s  VectorParamsAs1DForOutWhenUnconnected=off
  wires:
  Bias1/1 -> Switch/1
  Mod/1 -> Switch/2, Switch/3, Bias1/1
  Sum/1 -> Bias/1
  Bias/1 -> Mod/1
  Switch/1 -> timeToLatestUTCTimestamp/1
  Constant/1 -> Mod/2
  currentTimestampUTC/1 -> Sum/1
  latestTimestampUTC/1 -> Sum/2

== system GenericTarget/Time/UNIX Time ==
  SFunctionGTDriverUnixTime : S-Function  FunctionName=SFunctionGTDriverUnixTime  Parameters=SampleTime  SFunctionDeploymentMode=off  EnableBusSupport=off  mask(Legacy Function){SFunctionSpec=void GT_DriverUnixTimeStep(double y1[1]), SampleTime=SampleTime, ShowSpec=on}
      mask prompts: SampleTime "Sample time (-1 for inherited):"; ShowSpec "Display function specification"
      mask help:
      | This block allows you to call the legacy functions specified by the following Legacy Code Tool definition:
      | def.SFunctionName = 'SFunctionGTDriverUnixTime';
      | def.OutputFcnSpec = 'void GT_DriverUnixTimeStep(double y1[1])';
      | def.StartFcnSpec = 'void GT_DriverUnixTimeInitialize()';
      | def.TerminateFcnSpec = 'void GT_DriverUnixTimeTerminate()';
      | def.HeaderFiles = {'GT_DriverUnixTime.hpp'};
      | def.SourceFiles = {'GT_DriverUnixTime.cpp'};
      | def.SampleTime = 'parameterized';
      | def.Options.useTlcWithAccel = false;
      | def.Options.language = 'C++';
      mask Help: <p>This block was generated automatically by the Legacy Code Tool. For detailed help on this tool, call<a href="matlab:legacy_code('help')"> legacy_code('help')</a>.</p>
      mask Callback ShowSpec:
      | if strcmp(get_param(gcbh, 'ShowSpec'), 'on')
      |   set_param(gcbh, 'MaskDisplay', sprintf('fprintf(''%s'');', get_param(gcbh, 'SFunctionSpec')));
      | else
      |   set_param(gcbh, 'MaskDisplay', sprintf('fprintf(''%s'');', get_param(gcbh, 'FunctionName')));
      | end
      mask Display: fprintf('void GT_DriverUnixTimeStep(double y1[1])');
  time : Outport  OutDataTypeStr=double  Unit=s  PortDimensions=1  VectorParamsAs1DForOutWhenUnconnected=off
  wires:
  SFunctionGTDriverUnixTime/1 -> time/1

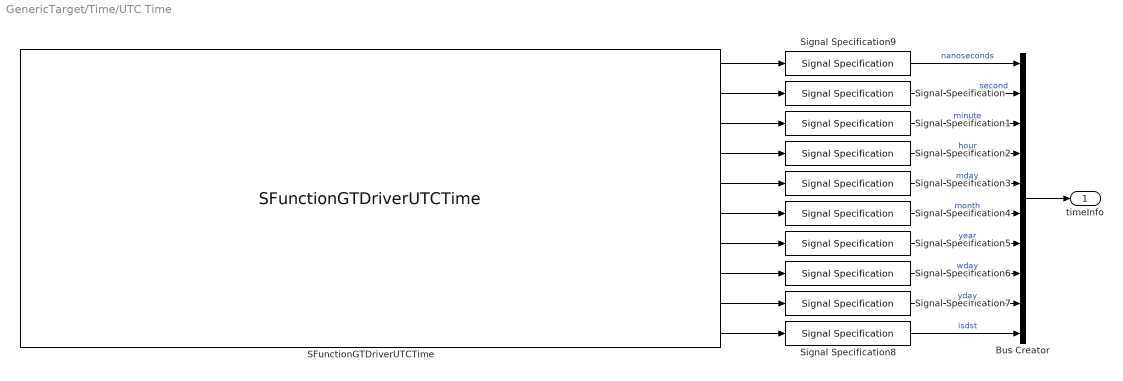
== system GenericTarget/Time/UTC Time ==
  Bus Creator : BusCreator  Inputs=10
  SFunctionGTDriverUTCTime : S-Function  FunctionName=SFunctionGTDriverUTCTime  Parameters=SampleTime  SFunctionDeploymentMode=off  EnableBusSupport=off  mask(Legacy Function){SFunctionSpec=void GT_DriverUTCTimeStep(int32 y1[1], int32 y2[1], int32 y3[1], int32 y4[1], int32 y5[1], int32 y6[1], int32 y7[1], int32 y8[1], int32 y9[1], int32 y10[1]), SampleTime=SampleTime, ShowSpec=on}
      mask prompts: SampleTime "Sample time (-1 for inherited):"; ShowSpec "Display function specification"
      mask help:
      | This block allows you to call the legacy functions specified by the following Legacy Code Tool definition:
      | def.SFunctionName = 'SFunctionGTDriverUTCTime';
      | def.OutputFcnSpec = 'void GT_DriverUTCTimeStep(int32 y1[1], int32 y2[1], int32 y3[1], int32 y4[1], int32 y5[1], int32 y6[1], int32 y7[1], int32 y8[1], int32 y9[1], int32 y10[1])';
      | def.StartFcnSpec = 'void GT_DriverUTCTimeInitialize()';
      | def.TerminateFcnSpec = 'void GT_DriverUTCTimeTerminate()';
      | def.HeaderFiles = {'GT_DriverUTCTime.hpp'};
      | def.SourceFiles = {'GT_DriverUTCTime.cpp'};
      | def.SampleTime = 'parameterized';
      | def.Options.useTlcWithAccel = false;
      | def.Options.language = 'C++';
      mask Help: <p>This block was generated automatically by the Legacy Code Tool. For detailed help on this tool, call<a href="matlab:legacy_code('help')"> legacy_code('help')</a>.</p>
      mask Callback ShowSpec:
      | if strcmp(get_param(gcbh, 'ShowSpec'), 'on')
      |   set_param(gcbh, 'MaskDisplay', sprintf('fprintf(''%s'');', get_param(gcbh, 'SFunctionSpec')));
      | else
      |   set_param(gcbh, 'MaskDisplay', sprintf('fprintf(''%s'');', get_param(gcbh, 'FunctionName')));
      | end
      mask Display: fprintf('void GT_DriverUTCTimeStep(int32 y1[1], int32 y2[1], int32 y3[1], int32 y4[1], int32 y5[1], int32 y6[1], int32 y7[1], int32 y8[1], int32 y9[1], int32 y10[1])');
  Signal Specification : SignalSpecification  OutDataTypeStr=int32  Unit=s  Dimensions=1
  Signal Specification1 : SignalSpecification  OutDataTypeStr=int32  Unit=min  Dimensions=1
  Signal Specification2 : SignalSpecification  OutDataTypeStr=int32  Unit=h  Dimensions=1
  Signal Specification3 : SignalSpecification  OutDataTypeStr=int32  Unit=d  Dimensions=1
  Signal Specification4 : SignalSpecification  OutDataTypeStr=int32  Dimensions=1
  Signal Specification5 : SignalSpecification  OutDataTypeStr=int32  Dimensions=1
  Signal Specification6 : SignalSpecification  OutDataTypeStr=int32  Unit=d  Dimensions=1
  Signal Specification7 : SignalSpecification  OutDataTypeStr=int32  Unit=d  Dimensions=1
  Signal Specification8 : SignalSpecification  OutDataTypeStr=int32  Dimensions=1
  Signal Specification9 : SignalSpecification  OutDataTypeStr=int32  Unit=ns  Dimensions=1
  timeInfo : Outport  VectorParamsAs1DForOutWhenUnconnected=off
  wires:
  Bus Creator/1 -> timeInfo/1
  Signal Specification/1 -> Bus Creator/2  "second"
  Signal Specification1/1 -> Bus Creator/3  "minute"
  Signal Specification2/1 -> Bus Creator/4  "hour"
  Signal Specification3/1 -> Bus Creator/5  "mday"
  Signal Specification4/1 -> Bus Creator/6  "month"
  Signal Specification5/1 -> Bus Creator/7  "year"
  Signal Specification6/1 -> Bus Creator/8  "wday"
  Signal Specification7/1 -> Bus Creator/9  "yday"
  Signal Specification8/1 -> Bus Creator/10  "isdst"
  SFunctionGTDriverUTCTime/1 -> Signal Specification9/1
  SFunctionGTDriverUTCTime/2 -> Signal Specification/1
  SFunctionGTDriverUTCTime/3 -> Signal Specification1/1
  SFunctionGTDriverUTCTime/4 -> Signal Specification2/1
  SFunctionGTDriverUTCTime/5 -> Signal Specification3/1
  SFunctionGTDriverUTCTime/6 -> Signal Specification4/1
  SFunctionGTDriverUTCTime/7 -> Signal Specification5/1
  SFunctionGTDriverUTCTime/8 -> Signal Specification6/1
  SFunctionGTDriverUTCTime/9 -> Signal Specification7/1
  SFunctionGTDriverUTCTime/10 -> Signal Specification8/1
  Signal Specification9/1 -> Bus Creator/1  "nanoseconds"

== system GenericTarget/Time/UTC Timestamp ==
  SFunctionGTDriverUTCTimestamp : S-Function  FunctionName=SFunctionGTDriverUTCTimestamp  Parameters=SampleTime  SFunctionDeploymentMode=off  EnableBusSupport=off  mask(Legacy Function){SFunctionSpec=void GT_DriverUTCTimestampStep(double y1[1]), SampleTime=SampleTime, ShowSpec=on}
      mask prompts: SampleTime "Sample time (-1 for inherited):"; ShowSpec "Display function specification"
      mask help:
      | This block allows you to call the legacy functions specified by the following Legacy Code Tool definition:
      | def.SFunctionName = 'SFunctionGTDriverUTCTimestamp';
      | def.OutputFcnSpec = 'void GT_DriverUTCTimestampStep(double y1[1])';
      | def.StartFcnSpec = 'void GT_DriverUTCTimestampInitialize()';
      | def.TerminateFcnSpec = 'void GT_DriverUTCTimestampTerminate()';
      | def.HeaderFiles = {'GT_DriverUTCTimestamp.hpp'};
      | def.SourceFiles = {'GT_DriverUTCTimestamp.cpp'};
      | def.SampleTime = 'parameterized';
      | def.Options.useTlcWithAccel = false;
      | def.Options.language = 'C++';
      mask Help: <p>This block was generated automatically by the Legacy Code Tool. For detailed help on this tool, call<a href="matlab:legacy_code('help')"> legacy_code('help')</a>.</p>
      mask Callback ShowSpec:
      | if strcmp(get_param(gcbh, 'ShowSpec'), 'on')
      |   set_param(gcbh, 'MaskDisplay', sprintf('fprintf(''%s'');', get_param(gcbh, 'SFunctionSpec')));
      | else
      |   set_param(gcbh, 'MaskDisplay', sprintf('fprintf(''%s'');', get_param(gcbh, 'FunctionName')));
      | end
      mask Display: fprintf('void GT_DriverUTCTimestampStep(double y1[1])');
  timestampUTC : Outport  OutDataTypeStr=double  Unit=s  PortDimensions=1  VectorParamsAs1DForOutWhenUnconnected=off
  wires:
  SFunctionGTDriverUTCTimestamp/1 -> timestampUTC/1

== system GenericTarget/Time/UTC Timestamp Moved On ==
  timestampUTC : Inport  OutDataTypeStr=double  Unit=s
  Compare To Zero : simulink/Logic and Bit Operations/Compare To Zero  relop=>  OutDataTypeStr=boolean
  Time To Latest UTC Timestamp : $bdroot/Time/Time To Latest UTC Timestamp
  Unit Delay : UnitDelay  InitialCondition=vinit  SampleTime=-1  HasFrameUpgradeWarning=on
  movedOn : Outport  OutDataTypeStr=boolean
  wires:
  timestampUTC/1 -> Unit Delay/1, Time To Latest UTC Timestamp/1
  Unit Delay/1 -> Time To Latest UTC Timestamp/2
  Time To Latest UTC Timestamp/1 -> Compare To Zero/1
  Compare To Zero/1 -> movedOn/1

== system GenericTarget/Examples/UDP Receive Loop/hold valid message ==
  In1 : Inport
  Enable : EnablePort
  Out1 : Outport
  wires:
  In1/1 -> Out1/1

== system GenericTarget/Interface/UDP Receive/atomic wrapper with sampletime ==
  groupBytes : Inport
  WhileIteratorSubsystem : Subsystem  TreatAsAtomicUnit=on
  bytes : Outport
  length : Outport  Port=2
  sourceAddress : Outport  Port=3
  sourcePort : Outport  Port=4
  result : Outport  Port=5
  lastErrorCode : Outport  Port=6
  wires:
  groupBytes/1 -> WhileIteratorSubsystem/1(groupBytes)
  WhileIteratorSubsystem/4(sourcePort) -> sourcePort/1
  WhileIteratorSubsystem/5(result) -> result/1
  WhileIteratorSubsystem/2(length) -> length/1
  WhileIteratorSubsystem/6(lastErrorCode) -> lastErrorCode/1
  WhileIteratorSubsystem/3(sourceAddress) -> sourceAddress/1
  WhileIteratorSubsystem/1(bytes) -> bytes/1
